simulink model "MCC_modek"  (R2025b)
settings: Solver=VariableStepAuto  StartTime=0.0  StopTime=4  RelTol=1e-3
undefined symbols (not defined in the file): cf, f, J, Ke, Kt, L, R, r
settings Model: Creator=liset  LastModifiedBy=liset

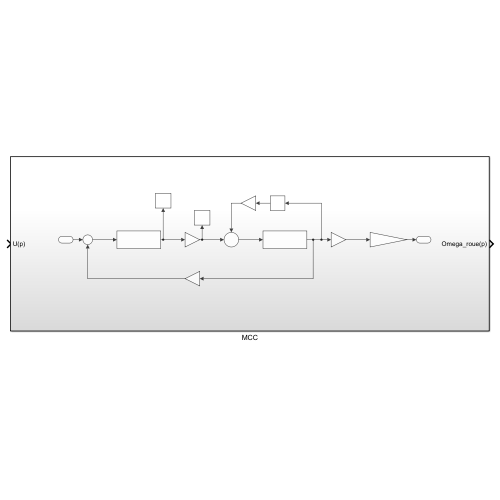
[thumbnail: Simulink's stored preview of the top-level diagram]
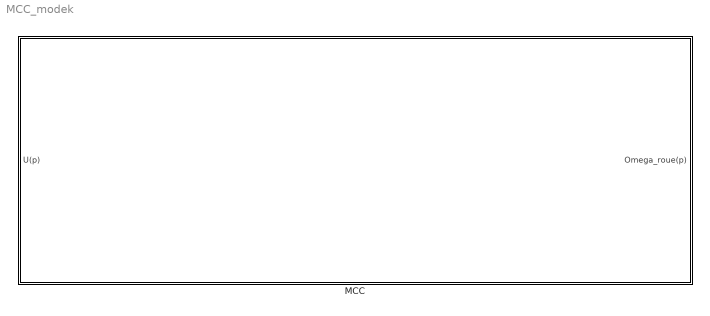
== system MCC_modek ==
  MCC : Subsystem

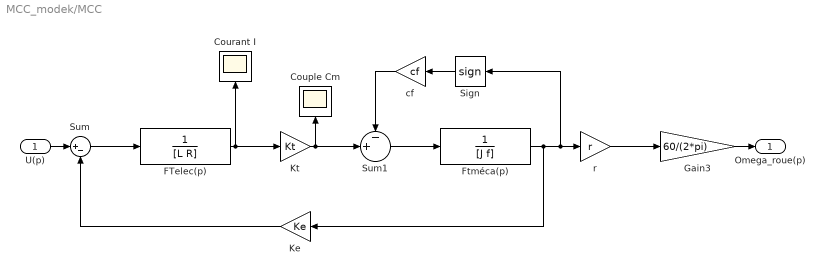
== system MCC_modek/MCC ==
  U(p) : Inport
  Couple Cm : Scope
      settings: ActiveDisplayYMinimum=-1  ActiveDisplayYMaximum=1  DataLoggingVariableName=ScopeData2
  Courant I : Scope
      settings: ActiveDisplayYMinimum=-1  ActiveDisplayYMaximum=1
  FTelec(p) : TransferFcn  Denominator=[L R]
  Ftméca(p) : TransferFcn  Denominator=[J f]
  Gain3 : Gain  Gain=60/(2*pi)
  Ke : Gain  Gain=Ke
  Kt : Gain  Gain=Kt
  Sign : Signum
  Sum : Sum  Inputs=|+-
  Sum1 : Sum  Inputs=-+|
  cf : Gain  Gain=cf
  r : Gain  Gain=r
  Omega_roue(p) : Outport
  wires:
  Sum1/1 -> Ftméca(p)/1
  Sum/1 -> FTelec(p)/1
  Kt/1 -> Couple Cm/1, Sum1/2
  r/1 -> Gain3/1
  Ftméca(p)/1 -> r/1, Sign/1, Ke/1
  FTelec(p)/1 -> Kt/1, Courant I/1
  Ke/1 -> Sum/2
  Sign/1 -> cf/1
  cf/1 -> Sum1/1
  Gain3/1 -> Omega_roue(p)/1
  U(p)/1 -> Sum/1
